simulink model "boost_sim"  (R2020a)
settings: Solver=VariableStepAuto  StartTime=0.0  StopTime=Inf  FixedStep=T  RelTol=1e-3
PostLoadFcn:
  | , if any(exist('dsrtsu_mdlpostloadfcn', 'file') ~= 0), dsrtsu_mdlpostloadfcn('Execute', bdroot); end,
InitFcn:
  | , if any(exist('rtifpga_mdlclblib', 'file') ~= 0), rtifpga_mdlclblib('Init', bdroot); end,
model workspace (MAT data in the model file):
  FPGA_boost_sim_1_Interrupt_1_1_write : Simulink.Signal (value not decoded)
  FPGA_boost_sim_1_Register_1_1_1_write : Simulink.Signal (value not decoded)
values from neighbouring files (symbols this model uses):
  fixedgain_i1 = 10*1000/(3*100)    (= 33.3333333333)    [param.m]
  fixedgain_v1 = 10*44000/(3*100*2.5)    (= 586.666666667)    [param.m]
  fixedgain_v2 = 10*10000/(3*100*2.5)    (= 133.333333333)    [param.m]
  gain_i1 = 1    [param.m]
  gain_v1 = 1    [param.m]
  gain_v2 = 1    [param.m]
  offset_i1 = .1    (= 0.1)    [param.m]
  offset_v1 = -10    [param.m]
  offset_v2 = 0    [param.m]
libraries: xbsIndex_r4 x39, rti1202lib_adc_class1 x3, rtiproclib x3, simulink x1, rtifpgainterfacelib x1
(part 3 of 3)

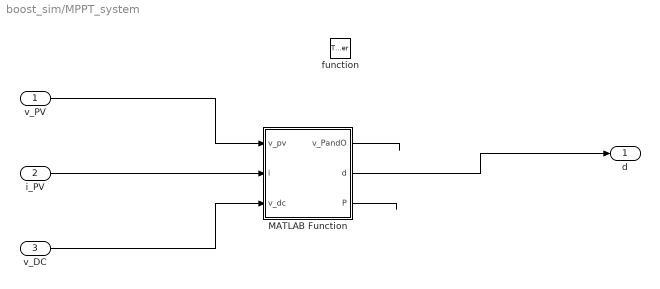
== system boost_sim/MPPT_system ==
  v_PV : Inport
  i_PV : Inport  Port=2
  v_DC : Inport  Port=3
  function : TriggerPort  TriggerType=function-call  VariantControl=Variant
  MATLAB Function : MATLAB Function  TreatAsAtomicUnit=on
  d : Outport
  wires:
  MATLAB Function/2(d) -> d/1
  i_PV/1 -> MATLAB Function/2(i)
  MATLAB Function/1(v_PandO) -> ?
  v_PV/1 -> MATLAB Function/1(v_pv)
  v_DC/1 -> MATLAB Function/3(v_dc)
  MATLAB Function/3(P) -> ?

== system boost_sim/RTI Data ==
  RTI Data Store : Subsystem  Tag="struct('private',struct('version',struct('dsVer',uint32(2)),'access',struct('modified',['20-Mar-2025 15:50:50'],'type','Model','isPerm',1)),'public',struct('main',struct('data',[]),'sub',struct('name',{{'boost_sim'}},'data',{{struct('TH',struct('thTaskInfo',struct('taskType',{'TIMER','HWINT','TMRINT','SWINT','GLINT'},'tasksNumOf',{1,1,0,0,0},'srcIds',{{'TIMERA'},{'FPGACL1FPGA_INTP0Ch0'},{},{},{}},'taskNames',{{['Timer Task 1']},{['PROC_INT_BL1 - interrupt']},{},{},{}})),'th_tc',struct('dataType',{'TASK','TASK'},'taskGroupId',{'',''},'taskGroupList',{{},{}},'taskSchedulingPolicy',{'FCFS','FCFS'},'taskType',{'TIMER','HWINT'},'blkh',{-1,['boost_sim/PROC_INT_BL1 - interrupt/Common Hardware' char(10) 'Interrupt Interface']},'srcId',{'TIMERA','FPGACL1FPGA_INTP0Ch0'},'srcSgnName',{['Timer A interrupt'],['FPGA Type CL1 FPGA_INT Port 0 Channel 0']},'srcCpuName',{'',''},'taskName',{['Timer Task 1  [5e-05] s'],['PROC_INT_BL1 - interrupt']},'taskNameDisplayExt',{'',''},'smplTime',{5e-5,0},'smplTimeOffs',{0,0},'hasFixedPriority',{0,0},'priority',{2,1},'hasFixedOvc',{0,0},'ovcType',{1,1},'ovcMax',{1,1}),'tc_th',struct('dataType',{'TASK','TASK'},'taskGroupId',{'',''},'taskGroupList',{{},{}},'taskSchedulingPolicy',{'FCFS','FCFS'},'taskType',{'TIMER','HWINT'},'blkh',{-1,['boost_sim/PROC_INT_BL1 - interrupt/Common Hardware' char(10) 'Interrupt Interface']},'srcId',{'TIMERA','FPGACL1FPGA_INTP0Ch0'},'srcSgnName',{['Timer A interrupt'],['FPGA Type CL1 FPGA_INT Port 0 Channel 0']},'srcCpuName',{'',''},'taskName',{['Timer Task 1  [5e-05] s'],['PROC_INT_BL1 - interrupt']},'taskNameDisplayExt',{'',''},'smplTime',{5e-5,0},'smplTimeOffs',{0,0},'hasFixedPriority',{0,0},'priority',{2,1},'hasFixedOvc',{0,0},'ovcType',{1,1},'ovcMax',{1,1}))}})))"  mask(RTI_DATA_STORE){}
      mask help:
      | RTI Data Store Block. This block is used by RTI to store internal model dependent data. Deleting this block will result in data loss.
      |
      | NEVER DELETE, COPY, OR MODIFY THIS BLOCK!
      mask Help:
      | RTI Data Store Block. This block is used by RTI to store internal model dependent data. Deleting this block will result in data loss.
      | 
      | NEVER DELETE, COPY, OR MODIFY THIS BLOCK!
      mask Display: text(0.5, 0.5, ' ', 'HorizontalAlignment', 'center');

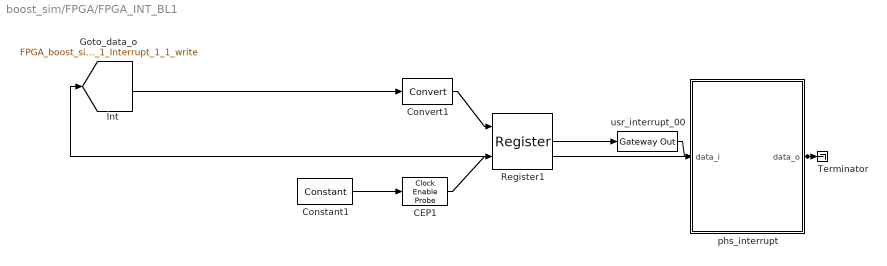
== system boost_sim/FPGA/FPGA_INT_BL1 ==
  Int : Inport
  CEP1 : xbsIndex_r4/Clock Enable Probe  inherit_constraints=off  block_type=ceprobe
      settings: infoedit="Clock enable extractor.  Produces a Boolean output that mirrors the hardware clock enable associated with the input sample rate.<br><br>Hardware notes: in hardware this block costs nothing."
  Constant1 : xbsIndex_r4/Constant  const=1  gui_display_data_type=Fixed-point  arith_type=Boolean  n_bits=16  bin_pt=14  preci_type=Single  exp_width=8  frac_width=24  explicit_period=on  period=1*1e-08  equ=P=C  opselect=C  inp2=PCIN>>17  opr=+  inp1=P  carry=CIN  dbl_ovrd=off  block_type=constant
  Convert1 : xbsIndex_r4/Convert  gui_display_data_type=Fixed-point  arith_type=Unsigned  n_bits=1  bin_pt=0  float_type=Single  exp_bits=8  fraction_bits=24  quantization=Truncate  overflow=Wrap  en=off  latency=0  pipeline=off  dbl_ovrd=off  block_type=convert
  Register1 : xbsIndex_r4/Register  init=0  rst=off  en=on  dbl_ovrd=off  block_type=register
  Terminator : Terminator
  phs_interrupt : Subsystem
  usr_interrupt_00 : xbsIndex_r4/Gateway Out  inherit_from_input=off  hdl_port=on  rows=1  columns=1  UseAsDAC=off  DACChannel='1'  interface=None  automatic_assignment=on  address_offset=hex2dec('00')  intf_name=''  intf_description=''  timing_constraint=None  locs_specified=off  LOCs={}  io_standard={}  block_type=gatewayout
  tag scope: FPGA_boost_sim_1_Interrupt_1_1_write=global
  wires:
  Constant1/1 -> CEP1/1
  CEP1/1 -> Register1/2
  Register1/1 -> usr_interrupt_00/1
  Int/1 -> Convert1/1
  Convert1/1 -> Register1/1
  usr_interrupt_00/1 -> phs_interrupt/1(data_i)
  phs_interrupt/1(data_o) -> Terminator/1, [FPGA_boost_sim_1_Interrupt_1_1_write]

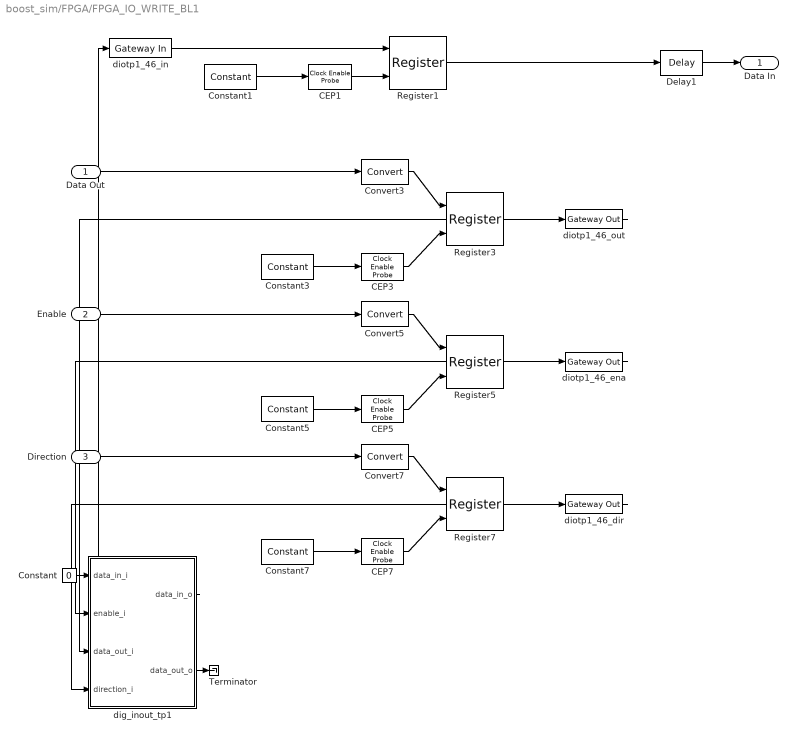
== system boost_sim/FPGA/FPGA_IO_WRITE_BL1 ==
  Data Out : Inport
  Enable : Inport  Port=2
  Direction : Inport  Port=3
  CEP{1,3,5,7} (4 alike) : xbsIndex_r4/Clock Enable Probe  inherit_constraints=off  block_type=ceprobe
      settings: infoedit="Clock enable extractor.  Produces a Boolean output that mirrors the hardware clock enable associated with the input sample rate.<br><br>Hardware notes: in hardware this block costs nothing."
  Constant : Constant  Value=0
  Constant{1,3,5,7} (4 alike) : xbsIndex_r4/Constant  const=1  gui_display_data_type=Fixed-point  arith_type=Boolean  n_bits=16  bin_pt=14  preci_type=Single  exp_width=8  frac_width=24  explicit_period=on  period=1*1e-08  equ=P=C  opselect=C  inp2=PCIN>>17  opr=+  inp1=P  carry=CIN  dbl_ovrd=off  block_type=constant
  Convert3 : xbsIndex_r4/Convert  gui_display_data_type=Fixed-point  arith_type=Unsigned  n_bits=1  bin_pt=0  float_type=Single  exp_bits=8  fraction_bits=24  quantization=Truncate  overflow=Wrap  en=off  latency=0  pipeline=off  dbl_ovrd=off  block_type=convert
  Convert5 : xbsIndex_r4/Convert  gui_display_data_type=Fixed-point  arith_type=Unsigned  n_bits=1  bin_pt=0  float_type=Single  exp_bits=8  fraction_bits=24  quantization=Truncate  overflow=Wrap  en=off  latency=0  pipeline=off  dbl_ovrd=off  block_type=convert
  Convert7 : xbsIndex_r4/Convert  gui_display_data_type=Fixed-point  arith_type=Unsigned  n_bits=1  bin_pt=0  float_type=Single  exp_bits=8  fraction_bits=24  quantization=Truncate  overflow=Wrap  en=off  latency=0  pipeline=off  dbl_ovrd=off  block_type=convert
  Delay1 : xbsIndex_r4/Delay  rst=off  infoeditControl=Selection of Reset will increase slice count due to use of real FFs and instead of SRLs  en=off  latency=0  reg_retiming=off  dbl_ovrd=off  block_type=delay
  Register{1,3,5,7} (4 alike) : xbsIndex_r4/Register  init=0  rst=off  en=on  dbl_ovrd=off  block_type=register
  Terminator : Terminator
  dig_inout_tp1 : Subsystem
      mask init:
      | par = rtifpgafcnlib('GetCurrentParaValue', get_param(get(gcbh, 'parent'), 'handle'));
      | if isempty(par)
      |     return
      | end
      | inverted_dio = str2double(par(2).Value{1});
      | vsetting = str2double(par(5).Value{1});
      | switch vsetting 
      |     case 1
      |         voltage = 3.3
      |     case 2
      |         voltage = 2.5;
      |     otherwise
      |         voltage = 5;
      | end
  diotp1_46_dir : xbsIndex_r4/Gateway Out  inherit_from_input=off  hdl_port=on  rows=1  columns=1  UseAsDAC=off  DACChannel='1'  interface=None  automatic_assignment=on  address_offset=hex2dec('00')  intf_name=''  intf_description=''  timing_constraint=None  locs_specified=off  LOCs={}  io_standard={}  block_type=gatewayout
  diotp1_46_ena : xbsIndex_r4/Gateway Out  inherit_from_input=off  hdl_port=on  rows=1  columns=1  UseAsDAC=off  DACChannel='1'  interface=None  automatic_assignment=on  address_offset=hex2dec('00')  intf_name=''  intf_description=''  timing_constraint=None  locs_specified=off  LOCs={}  io_standard={}  block_type=gatewayout
  diotp1_46_in : xbsIndex_r4/Gateway In  gui_display_data_type=Fixed-point  arith_type=Unsigned  n_bits=1  bin_pt=0  preci_type=Single  exp_width=8  frac_width=24  rows=1  columns=1  quantization="Round  (unbiased: +/- Inf)"  overflow=Saturate  period=1e-08  UseAsADC=off  ADCChannel='1'  interface=None  automatic_assignment=on  address_offset=hex2dec('00')  intf_name=''  intf_description=''  default_value=0  timing_constraint=None  locs_specified=off  LOCs={}  io_standard={}  inherit_from_input=off  hdl_port=on  dbl_ovrd=off  block_type=gatewayin
  diotp1_46_out : xbsIndex_r4/Gateway Out  inherit_from_input=off  hdl_port=on  rows=1  columns=1  UseAsDAC=off  DACChannel='1'  interface=None  automatic_assignment=on  address_offset=hex2dec('00')  intf_name=''  intf_description=''  timing_constraint=None  locs_specified=off  LOCs={}  io_standard={}  block_type=gatewayout
  Data In : Outport
  wires:
  Register1/1 -> Delay1/1
  Delay1/1 -> Data In/1
  Constant1/1 -> CEP1/1
  CEP1/1 -> Register1/2
  diotp1_46_in/1 -> Register1/1
  Constant3/1 -> CEP3/1
  CEP3/1 -> Register3/2
  Register3/1 -> diotp1_46_out/1
  Data Out/1 -> Convert3/1
  Convert3/1 -> Register3/1
  Constant5/1 -> CEP5/1
  CEP5/1 -> Register5/2
  Register5/1 -> diotp1_46_ena/1
  Enable/1 -> Convert5/1
  Convert5/1 -> Register5/1
  Constant7/1 -> CEP7/1
  CEP7/1 -> Register7/2
  Register7/1 -> diotp1_46_dir/1
  Direction/1 -> Convert7/1
  Convert7/1 -> Register7/1
  dig_inout_tp1/1(data_in_o) -> diotp1_46_in/1
  diotp1_46_out/1 -> dig_inout_tp1/3(data_out_i)
  diotp1_46_ena/1 -> dig_inout_tp1/2(enable_i)
  diotp1_46_dir/1 -> dig_inout_tp1/4(direction_i)
  Constant/1 -> dig_inout_tp1/1(data_in_i)
  dig_inout_tp1/2(data_out_o) -> Terminator/1

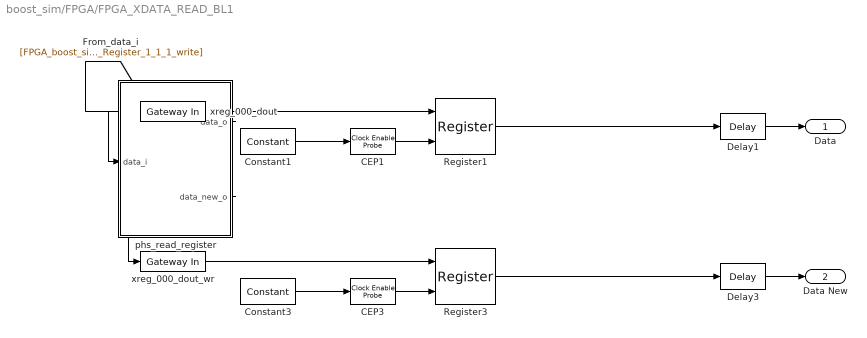
== system boost_sim/FPGA/FPGA_XDATA_READ_BL1 ==
  CEP1 : xbsIndex_r4/Clock Enable Probe  inherit_constraints=off  block_type=ceprobe
      settings: infoedit="Clock enable extractor.  Produces a Boolean output that mirrors the hardware clock enable associated with the input sample rate.<br><br>Hardware notes: in hardware this block costs nothing."
  CEP3 : xbsIndex_r4/Clock Enable Probe  inherit_constraints=off  block_type=ceprobe
      settings: infoedit="Clock enable extractor.  Produces a Boolean output that mirrors the hardware clock enable associated with the input sample rate.<br><br>Hardware notes: in hardware this block costs nothing."
  Constant1 : xbsIndex_r4/Constant  const=1  gui_display_data_type=Fixed-point  arith_type=Boolean  n_bits=16  bin_pt=14  preci_type=Single  exp_width=8  frac_width=24  explicit_period=on  period=1*1e-08  equ=P=C  opselect=C  inp2=PCIN>>17  opr=+  inp1=P  carry=CIN  dbl_ovrd=off  block_type=constant
  Constant3 : xbsIndex_r4/Constant  const=1  gui_display_data_type=Fixed-point  arith_type=Boolean  n_bits=16  bin_pt=14  preci_type=Single  exp_width=8  frac_width=24  explicit_period=on  period=1*1e-08  equ=P=C  opselect=C  inp2=PCIN>>17  opr=+  inp1=P  carry=CIN  dbl_ovrd=off  block_type=constant
  Delay1 : xbsIndex_r4/Delay  rst=off  infoeditControl=Selection of Reset will increase slice count due to use of real FFs and instead of SRLs  en=off  latency=0  reg_retiming=off  dbl_ovrd=off  block_type=delay
  Delay3 : xbsIndex_r4/Delay  rst=off  infoeditControl=Selection of Reset will increase slice count due to use of real FFs and instead of SRLs  en=off  latency=0  reg_retiming=off  dbl_ovrd=off  block_type=delay
  Register1 : xbsIndex_r4/Register  init=0  rst=off  en=on  dbl_ovrd=off  block_type=register
  Register3 : xbsIndex_r4/Register  init=0  rst=off  en=on  dbl_ovrd=off  block_type=register
  phs_read_register : Subsystem
      mask init:
      | [par, fct] = rtifpgafcnlib('GetCurrentParaValue', get_param(get(gcbh, 'parent'), 'handle'), 'all');
      | if isempty(par) || isempty(fct)
      |     return
      | end
      | binaryPoint = str2double(par(1).Value{1});
      | format = par(2).Value{1};
      | if (strcmp(format, 'signed') == 1)
      |     mode = 0;
      | elseif (strcmp(format, 'unsigned') == 1)
      |     mode = 1;
      | else
      |     % floating-point
      |     mode = 2;
      | end
      | 
      | %Determine PROC sample time
      | proc_sample_time_field = par(5).Value{1};
      | num_val = str2num(proc_sample_time_field);
      | if ~isempty(num_val)
      |     proc_sample_time = num_val;
      | else % search for subsystem/workspace value
      |     proc_sample_time = rtifpgafcnlib('SearchVariableValue', gcbh, proc_sample_time_field);
      |     if ~isnumeric(proc_sample_time)
      |         proc_sample_time = str2double(proc_sample_time);
      |     end
      | end
      | 
      | %Determine FPGA sample rate
      | dataGatewayName = fct.FrameworkIn(1).Name{1};
      | fpga_sample_time = rtifpga_xsgcasinglib('xlGetParam', [gcs '/' dataGatewayName] , 'period');
      | fpga_sample_time = str2double(fpga_sample_time);
  xreg_000_dout : xbsIndex_r4/Gateway In  gui_display_data_type=Fixed-point  arith_type=Unsigned  n_bits=32  bin_pt=0  preci_type=Single  exp_width=8  frac_width=24  rows=1  columns=1  quantization="Round  (unbiased: +/- Inf)"  overflow=Saturate  period=1e-08  UseAsADC=off  ADCChannel='1'  interface=None  automatic_assignment=on  address_offset=hex2dec('00')  intf_name=''  intf_description=''  default_value=0  timing_constraint=None  locs_specified=off  LOCs={}  io_standard={}  inherit_from_input=off  hdl_port=on  dbl_ovrd=off  block_type=gatewayin
  xreg_000_dout_wr : xbsIndex_r4/Gateway In  gui_display_data_type=Fixed-point  arith_type=Unsigned  n_bits=1  bin_pt=0  preci_type=Single  exp_width=8  frac_width=24  rows=1  columns=1  quantization="Round  (unbiased: +/- Inf)"  overflow=Saturate  period=1e-08  UseAsADC=off  ADCChannel='1'  interface=None  automatic_assignment=on  address_offset=hex2dec('00')  intf_name=''  intf_description=''  default_value=0  timing_constraint=None  locs_specified=off  LOCs={}  io_standard={}  inherit_from_input=off  hdl_port=on  dbl_ovrd=off  block_type=gatewayin
  Data : Outport
  Data New : Outport  Port=2
  wires:
  Register1/1 -> Delay1/1
  Delay1/1 -> Data/1
  Constant1/1 -> CEP1/1
  CEP1/1 -> Register1/2
  xreg_000_dout/1 -> Register1/1
  Register3/1 -> Delay3/1
  Delay3/1 -> Data New/1
  Constant3/1 -> CEP3/1
  CEP3/1 -> Register3/2
  xreg_000_dout_wr/1 -> Register3/1
  phs_read_register/1(data_o) -> xreg_000_dout/1
  phs_read_register/2(data_new_o) -> xreg_000_dout_wr/1
  [FPGA_boost_sim_1_Register_1_1_1_write] -> phs_read_register/1(data_i)

== system boost_sim/RTI Data/RTI Data Store ==
  RTI Data Store : Subsystem  mask(RTI_DATA_STORE){}
      mask help:
      | RTI Data Store Block. This block is used by RTI to store internal model dependent data. Deleting this block will result in data loss.
      |
      | NEVER DELETE, COPY, OR MODIFY THIS BLOCK!
      mask Help:
      | RTI Data Store Block. This block is used by RTI to store internal model dependent data. Deleting this block will result in data loss.
      | 
      | NEVER DELETE, COPY, OR MODIFY THIS BLOCK!
      mask Display: text(0.5, 0.5, ' ', 'HorizontalAlignment', 'center');

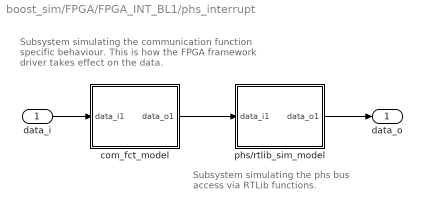
== system boost_sim/FPGA/FPGA_INT_BL1/phs_interrupt ==
  note: Subsystem simulating the phs bus
      | access via RTLib functions.
  note: Subsystem simulating the communication
      | function specific behaviour. This is how the
      | FPGA framework driver takes effect on the data.
  data_i : Inport
  com_fct_model : Subsystem
  phs/rtlib_sim_model : Subsystem
  data_o : Outport  VectorParamsAs1DForOutWhenUnconnected=off
  wires:
  phs/rtlib_sim_model/1(data_o1) -> data_o/1
  com_fct_model/1(data_o1) -> phs/rtlib_sim_model/1(data_i1)
  data_i/1 -> com_fct_model/1(data_i1)

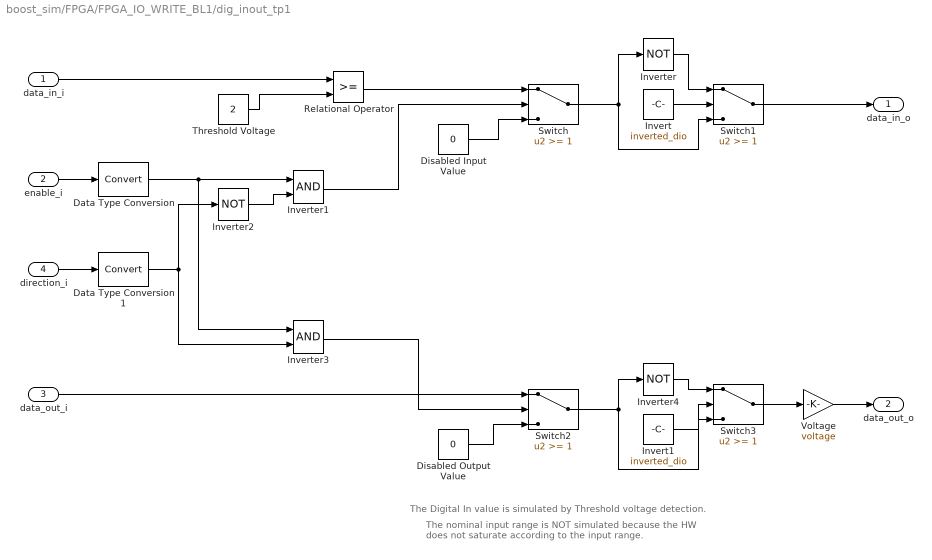
== system boost_sim/FPGA/FPGA_IO_WRITE_BL1/dig_inout_tp1 ==
  note: The nominal input range is NOT simulated because
      | the HW does not saturate according to the input range.
  note: The Digital In value is simulated by Threshold voltage detection.
  data_in_i : Inport
  enable_i : Inport  Port=2
  data_out_i : Inport  Port=3
  direction_i : Inport  Port=4
  Data Type Conversion : DataTypeConversion
  Data Type Conversion1 : DataTypeConversion
  Disabled Input Value : Constant  Value=0
  Disabled Output Value : Constant  Value=0
  Invert : Constant  Value=inverted_dio
  Invert1 : Constant  Value=inverted_dio
  Inverter : Logic  Operator=NOT  AllPortsSameDT=off  OutDataTypeStr=boolean
  Inverter1 : Logic  AllPortsSameDT=off  OutDataTypeStr=boolean
  Inverter2 : Logic  Operator=NOT  AllPortsSameDT=off  OutDataTypeStr=boolean
  Inverter3 : Logic  AllPortsSameDT=off  OutDataTypeStr=boolean
  Inverter4 : Logic  Operator=NOT  AllPortsSameDT=off  OutDataTypeStr=boolean
  Relational Operator : RelationalOperator  OutDataTypeStr=boolean  RndMeth=Nearest
  Switch{,1..3} (4 alike) : Switch  Threshold=1
  Threshold Voltage : Constant  Value=2
  Voltage : Gain  Gain=voltage  ParamDataTypeStr=float('double')
  data_in_o : Outport  VectorParamsAs1DForOutWhenUnconnected=off
  data_out_o : Outport  Port=2  VectorParamsAs1DForOutWhenUnconnected=off
  wires:
  Voltage/1 -> data_out_o/1
  Data Type Conversion1/1 -> Inverter3/2, Inverter2/1
  Data Type Conversion/1 -> Inverter3/1, Inverter1/1
  Switch3/1 -> Voltage/1
  Switch2/1 -> Switch3/3, Inverter4/1
  Inverter4/1 -> Switch3/1
  Invert1/1 -> Switch3/2
  data_out_i/1 -> Switch2/1
  Inverter3/1 -> Switch2/2
  Disabled Output Value/1 -> Switch2/3
  Inverter2/1 -> Inverter1/2
  direction_i/1 -> Data Type Conversion1/1
  Inverter1/1 -> Switch/2
  enable_i/1 -> Data Type Conversion/1
  Switch/1 -> Switch1/3, Inverter/1
  Relational Operator/1 -> Switch/1
  Inverter/1 -> Switch1/1
  Invert/1 -> Switch1/2
  Switch1/1 -> data_in_o/1
  Disabled Input Value/1 -> Switch/3
  Threshold Voltage/1 -> Relational Operator/2
  data_in_i/1 -> Relational Operator/1

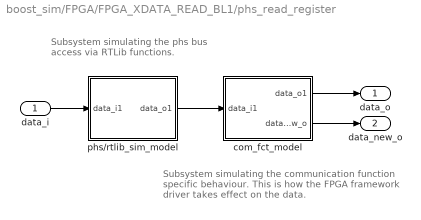
== system boost_sim/FPGA/FPGA_XDATA_READ_BL1/phs_read_register ==
  note: Subsystem simulating the phs bus
      | access via RTLib functions.
  note: Subsystem simulating the communication
      | function specific behaviour. This is how the
      | FPGA framework driver takes effect on the data.
  data_i : Inport
  com_fct_model : Subsystem
  phs/rtlib_sim_model : Subsystem
  data_o : Outport  VectorParamsAs1DForOutWhenUnconnected=off
  data_new_o : Outport  Port=2  VectorParamsAs1DForOutWhenUnconnected=off
  wires:
  com_fct_model/2(data_new_o) -> data_new_o/1
  phs/rtlib_sim_model/1(data_o1) -> com_fct_model/1(data_i1)
  com_fct_model/1(data_o1) -> data_o/1
  data_i/1 -> phs/rtlib_sim_model/1(data_i1)

== system boost_sim/RTI Data/RTI Data Store/RTI Data Store ==
  RTI Data Store : Subsystem  mask(RTI_DATA_STORE){}
      mask help:
      | RTI Data Store Block. This block is used by RTI to store internal model dependent data. Deleting this block will result in data loss.
      |
      | NEVER DELETE, COPY, OR MODIFY THIS BLOCK!
      mask Help:
      | RTI Data Store Block. This block is used by RTI to store internal model dependent data. Deleting this block will result in data loss.
      | 
      | NEVER DELETE, COPY, OR MODIFY THIS BLOCK!
      mask Display: text(0.5, 0.5, ' ', 'HorizontalAlignment', 'center');

== system boost_sim/FPGA/FPGA_INT_BL1/phs_interrupt/com_fct_model ==
  data_i1 : Inport
  data_o1 : Outport  VectorParamsAs1DForOutWhenUnconnected=off
  wires:
  data_i1/1 -> data_o1/1

== system boost_sim/FPGA/FPGA_INT_BL1/phs_interrupt/phs//rtlib_sim_model ==
  note: - Detect the interrupt (rising edge).
      | - Generate function call.
  data_i1 : Inport
  Triggered Subsystem : Subsystem  TreatAsAtomicUnit=on
  data_o1 : Outport  VectorParamsAs1DForOutWhenUnconnected=off
  wires:
  Triggered Subsystem/1(Out1) -> data_o1/1
  data_i1/1 -> Triggered Subsystem/Trigger

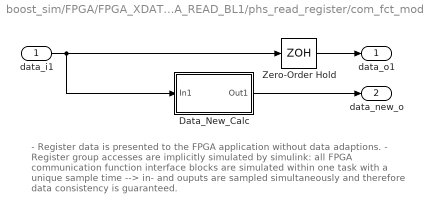
== system boost_sim/FPGA/FPGA_XDATA_READ_BL1/phs_read_register/com_fct_model ==
  note: - Register data is presented to the FPGA application without data adaptions.
      |
      | - Register group accesses are implicitly simulated by simulink: all FPGA
      | communication function interface blocks are simulated within one task
      | with a unique sample time --> in- and ouputs are sampled simultaneously
      | and therefore data consistency is guaranteed.
  data_i1 : Inport
  Data_New_Calc : Subsystem
  Zero-Order Hold : ZeroOrderHold  SampleTime=fpga_sample_time
  data_o1 : Outport  VectorParamsAs1DForOutWhenUnconnected=off
  data_new_o : Outport  Port=2  VectorParamsAs1DForOutWhenUnconnected=off
  wires:
  Zero-Order Hold/1 -> data_o1/1
  Data_New_Calc/1(Out1) -> data_new_o/1
  data_i1/1 -> Zero-Order Hold/1, Data_New_Calc/1(In1)

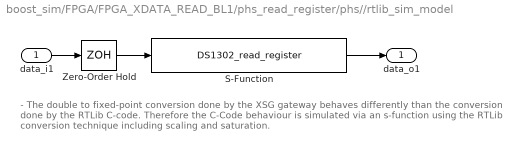
== system boost_sim/FPGA/FPGA_XDATA_READ_BL1/phs_read_register/phs//rtlib_sim_model ==
  note: - The double to fixed-point conversion done by the XSG gateway behaves differently
      | than the conversion done by the RTLib C-code. Therefore the C-Code behaviour
      | is simulated via an s-function using the RTLib conversion technique including scaling and saturation.
  data_i1 : Inport
  S-Function : S-Function  FunctionName=DS1302_read_register  Parameters=mode;binaryPoint  SFunctionDeploymentMode=off  EnableBusSupport=off
  Zero-Order Hold : ZeroOrderHold  SampleTime=proc_sample_time
  data_o1 : Outport  VectorParamsAs1DForOutWhenUnconnected=off
  wires:
  Zero-Order Hold/1 -> S-Function/1
  S-Function/1 -> data_o1/1
  data_i1/1 -> Zero-Order Hold/1

== system boost_sim/RTI Data/RTI Data Store/RTI Data Store/RTI Data Store ==
  RTI Data Store : Subsystem  mask(RTI_DATA_STORE){}
      mask help:
      | RTI Data Store Block. This block is used by RTI to store internal model dependent data. Deleting this block will result in data loss.
      |
      | NEVER DELETE, COPY, OR MODIFY THIS BLOCK!
      mask Help:
      | RTI Data Store Block. This block is used by RTI to store internal model dependent data. Deleting this block will result in data loss.
      | 
      | NEVER DELETE, COPY, OR MODIFY THIS BLOCK!
      mask Display: text(0.5, 0.5, ' ', 'HorizontalAlignment', 'center');

== system boost_sim/FPGA/FPGA_INT_BL1/phs_interrupt/phs//rtlib_sim_model/Triggered Subsystem ==
  Trigger : TriggerPort  VariantControl=(inherit)
  Function-Call Generator : simulink/Ports & Subsystems/Function-Call Generator  sample_time=-1  numberOfIterations=1
  Out1 : Outport  VectorParamsAs1DForOutWhenUnconnected=off
  wires:
  Function-Call Generator/1 -> Out1/1

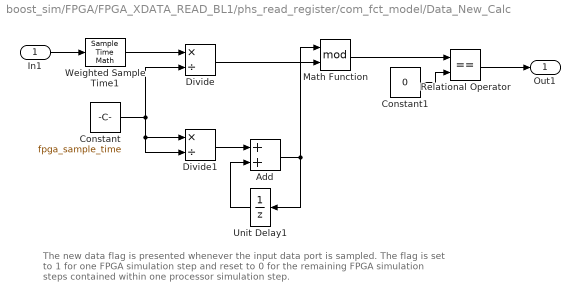
== system boost_sim/FPGA/FPGA_XDATA_READ_BL1/phs_read_register/com_fct_model/Data_New_Calc ==
  note: The new data flag is presented whenever the input data port is sampled.
      | The flag is set to 1 for one FPGA simulation step and reset to 0 for the
      | remaining FPGA simulation steps contained within one processor simulation step.
  In1 : Inport
  Add : Sum
  Constant : Constant  Value=fpga_sample_time  SampleTime=fpga_sample_time
  Constant1 : Constant  Value=0
  Divide : Product  Inputs=*/
  Divide1 : Product  Inputs=*/
  Math Function : Math  Operator=mod  SignedPower=on  SaturateOnIntegerOverflow=on
  Relational Operator : RelationalOperator  Operator===  OutDataTypeStr=boolean  RndMeth=Nearest
  Unit Delay1 : UnitDelay  InitialCondition=-1  SampleTime=-1  HasFrameUpgradeWarning=on
  Weighted Sample Time1 : SampleTimeMath  TsampMathOp=Ts Only
  Out1 : Outport  VectorParamsAs1DForOutWhenUnconnected=off
  wires:
  Constant/1 -> Divide1/2, Divide1/1, Divide/2
  Weighted Sample Time1/1 -> Divide/1
  Math Function/1 -> Relational Operator/1
  Relational Operator/1 -> Out1/1
  In1/1 -> Weighted Sample Time1/1
  Divide1/1 -> Add/1
  Unit Delay1/1 -> Add/2
  Add/1 -> Unit Delay1/1, Math Function/1
  Constant1/1 -> Relational Operator/2
  Divide/1 -> Math Function/2

== system boost_sim/RTI Data/RTI Data Store/RTI Data Store/RTI Data Store/RTI Data Store ==

== matlab function boost_sim/MPPT_system/MATLAB Function ==
  data: v_pv input; v_PandO output; i input; v_dc input; d output; P output
function [v_PandO, d, P] = MPPT(v_pv,i, v_dc)
persistent P_ant v_ref v_ant v_dc_ant

if isempty(P_ant)
    P_ant = 0;
    v_ref = 10;
    v_ant = 10;
end


P = v_pv*i;

v_dc_ant = v_dc;
delta = P-P_ant;

if (abs(delta) < 0.001)
elseif delta > 0
        if v_pv>v_ant
            v_ref = v_ref+.1;
        else
            v_ref = v_ref-.1;
        end
else
        if v_pv>v_ant
            v_ref = v_ref-.1;
        else
            v_ref = v_ref+.1;
        end
end
if v_ref>15
    v_ref = 15;
end
if v_ref<0
    v_ref = 0;
end
P_ant = P;
v_ant = v_pv;

v_PandO = v_ref;


g = v_dc_ant/v_ref;
d = 100*(1-(1/g)); %debe coincidir con el PWM de la FPGA (no el de interrupcion)
if d<2
    d = 2;
elseif d>98
    d=98;
end
